simulink model "AOOR"  (R2020a)
settings: Solver=FixedStepAuto  StartTime=0.0  StopTime=60  FixedStep=1e-3  RelTol=1e-3  EnableMultiTasking=on
undefined symbols (not defined in the file): D10, D11, D12, D2, D4, D5, D7, D8, D9, PTA0, PTA2, PTB23, PTB9, PTC3, PTC4, PTD0, PTD2, PTD3
libraries: frdmk64flib x11, dspstat3 x1
settings Model: ExtModeTrigDuration=5  Creator=raymo  LastModifiedBy=raymo
settings OptimizationCC: EnhancedBackFolding=on  PassReuseOutputArgsAs=Individual arguments  ZeroExternalMemoryAtStartup=off  ZeroInternalMemoryAtStartup=off  MaxStackSize=64  OptimizeBlockOrder=speed  DifferentSizesBufferReuse=on  OptimizationCustomize=off  EfficientTunableParamExpr=on
settings DebuggingCC: ParameterTunabilityLossMsg=error
settings HardwareCC: ProdBitPerPointer=32  ProdBitPerSizeT=32  ProdBitPerPtrDiffT=32  ProdLargestAtomicInteger=Long  ProdLargestAtomicFloat=Double  ProdWordSize=32  ProdHWDeviceType=ARM Compatible->ARM Cortex
settings SFSimCC: MATLABDynamicMemAlloc=off
settings RTWCC: SystemTargetFile=ert.tlc  HardwareBoard=NXP FRDM-K64F  TemplateMakefile=ert_default_tmf  Toolchain=GNU Tools for ARM Embedded Processors
settings CodeAppCC: ForceParamTrailComments=on  IgnoreCustomStorageClasses=off  OperatorAnnotations=on  SimulinkDataObjDesc=on  SFDataObjDesc=on  InsertBlockDesc=on

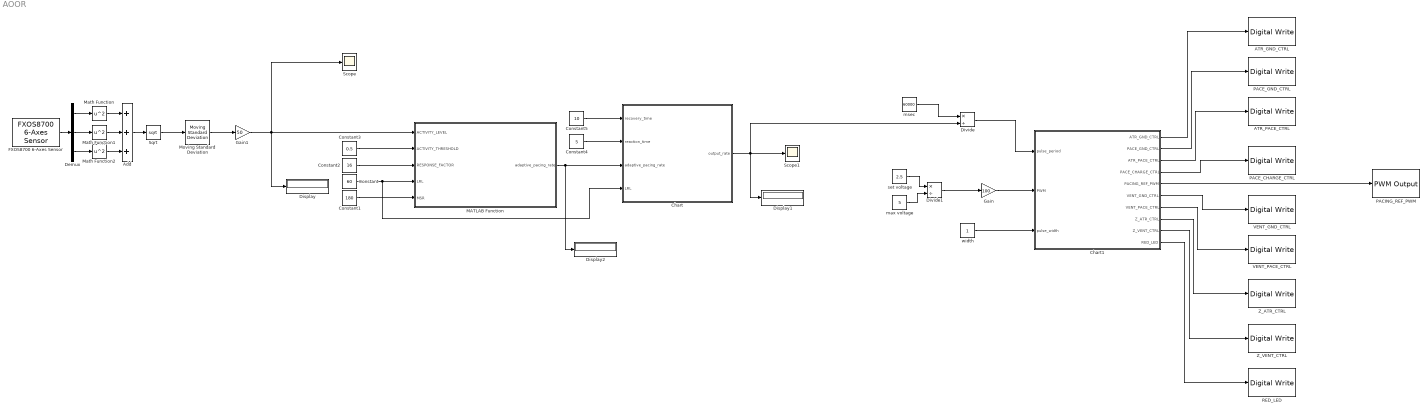
== system AOOR ==
  ATR_GND_CTRL : frdmk64flib/Digital Write  Whichpin=PTD2 (D11)
  ATR_PACE_CTRL : frdmk64flib/Digital Write  Whichpin=PTA0 (D8)
  Add : Sum  Inputs=+++
  Chart : Stateflow chart  TreatAsAtomicUnit=on
  Chart1 : Stateflow chart  TreatAsAtomicUnit=on
  Constant : Constant  Value=60
  Constant1 : Constant  Value=180
  Constant2 : Constant  Value=16
  Constant3 : Constant  Value=0.5
  Constant4 : Constant  Value=5
  Constant5 : Constant  Value=10
  Demux : Demux  Outputs=3
  Display : Display
  Display1 : Display
  Display2 : Display
  Divide : Product  Inputs=*/
  Divide1 : Product  Inputs=*/
  FXOS8700 6-Axes Sensor : frdmk64flib/FXOS8700 6-Axes Sensor  Activesensor=Accelerometer only  ODR=800Hz  HybridODR=400Hz  Accelfullrange=-4g to +4g  SampleTime=-1
  Gain : Gain  Gain=100
  Gain1 : Gain  Gain=50
  MATLAB Function : MATLAB Function  TreatAsAtomicUnit=on
  Math Function : Math  Operator=square  SaturateOnIntegerOverflow=on
  Math Function1 : Math  Operator=square  SaturateOnIntegerOverflow=on
  Math Function2 : Math  Operator=square  SaturateOnIntegerOverflow=on
  Moving Standard Deviation : dspstat3/Moving Standard Deviation  Method=Sliding window  ForgettingFactorPort=off  SpecifyWindowLength=on  WindowLength=4  ForgettingFactor=0.9  SimulateUsing=Code generation
      settings: SourceProductBaseCode=DS
  PACE_CHARGE_CTRL : frdmk64flib/Digital Write  Whichpin=PTB9 (D2)
  PACE_GND_CTRL : frdmk64flib/Digital Write  Whichpin=PTD0 (D10)
  PACING_REF_PWM : frdmk64flib/PWM Output  Whichpin=PTA2 (D5)  InitialFrequency=2000  InitialDutyCycle=50
  RED_LED : frdmk64flib/Digital Write  Whichpin=RED_LED
  Scope : Scope
  Scope1 : Scope
  Sqrt : Sqrt  SaturateOnIntegerOverflow=on
  VENT_GND_CTRL : frdmk64flib/Digital Write  Whichpin=PTD3 (D12)
  VENT_PACE_CTRL : frdmk64flib/Digital Write  Whichpin=PTC4 (D9)
  Z_ATR_CTRL : frdmk64flib/Digital Write  Whichpin=PTB23 (D4)
  Z_VENT_CTRL : frdmk64flib/Digital Write  Whichpin=PTC3 (D7)
  max voltage : Constant  Value=5
  msec : Constant  Value=60000
  set voltage : Constant  Value=2.5
  width : Constant
  wires:
  Math Function1/1 -> Add/2
  Add/1 -> Sqrt/1
  Demux/1 -> Math Function/1
  Demux/3 -> Math Function2/1
  Math Function2/1 -> Add/3
  Sqrt/1 -> Moving Standard Deviation/1
  Math Function/1 -> Add/1
  Demux/2 -> Math Function1/1
  FXOS8700 6-Axes Sensor/1 -> Demux/1
  MATLAB Function/1(adaptive_pacing_rate) -> Chart/3(adaptive_pacing_rate), Display2/1
  Constant/1 -> Chart/4(LRL), MATLAB Function/4(LRL)
  Constant1/1 -> MATLAB Function/5(MSR)
  Constant2/1 -> MATLAB Function/3(RESPONSE_FACTOR)
  Constant3/1 -> MATLAB Function/2(ACTIVITY_THRESHOLD)
  Constant5/1 -> Chart/1(recovery_time)
  Constant4/1 -> Chart/2(reaction_time)
  Chart/1(output_rate) -> Divide/2, Display1/1, Scope1/1
  Divide/1 -> Chart1/1(pulse_period)
  set voltage/1 -> Divide1/1
  Chart1/9(Z_VENT_CTRL) -> Z_VENT_CTRL/1
  Chart1/1(ATR_GND_CTRL) -> ATR_GND_CTRL/1
  Chart1/10(RED_LED) -> RED_LED/1
  width/1 -> Chart1/3(pulse_width)
  Chart1/3(ATR_PACE_CTRL) -> ATR_PACE_CTRL/1
  msec/1 -> Divide/1
  Chart1/4(PACE_CHARGE_CTRL) -> PACE_CHARGE_CTRL/1
  Chart1/6(VENT_GND_CTRL) -> VENT_GND_CTRL/1
  max voltage/1 -> Divide1/2
  Chart1/5(PACING_REF_PWM) -> PACING_REF_PWM/1
  Gain/1 -> Chart1/2(PWM)
  Chart1/7(VENT_PACE_CTRL) -> VENT_PACE_CTRL/1
  Chart1/8(Z_ATR_CTRL) -> Z_ATR_CTRL/1
  Divide1/1 -> Gain/1
  Chart1/2(PACE_GND_CTRL) -> PACE_GND_CTRL/1
  Moving Standard Deviation/1 -> Gain1/1
  Gain1/1 -> Scope/1, Display/1, MATLAB Function/1(ACTIVITY_LEVEL)

== stateflow chart AOOR/Chart1 ==
  state ChargeDishcharge
    entry:
    %C22
    ATR_PACE_CTRL = false;
    VENT_PACE_CTRL = false;
    PACING_REF_PWM = PWM;
    PACE_CHARGE_CTRL = true;
    %C21
    PACE_GND_CTRL = true;
    VENT_PACE_CTRL = false;
    Z_ATR_CTRL = false;
    Z_VENT_CTRL = false;
    ATR_GND_CTRL = true;
    VENT_GND_CTRL = false;
    %RED LED
    RED_LED = false;
  state AVpacing
    entry:
    PACE_CHARGE_CTRL = false;
    PACE_GND_CTRL = true;
    ATR_PACE_CTRL = true;
    ATR_GND_CTRL = false;
    Z_ATR_CTRL = false;
    Z_VENT_CTRL = false;
    VENT_GND_CTRL = false;
    VENT_PACE_CTRL = false;
    PACING_REF_PWM = PWM;
    RED_LED = true;
  (default) -> ChargeDishcharge
  AVpacing -> ChargeDishcharge : [after(pulse_width, msec)]
  ChargeDishcharge -> AVpacing : [after(pulse_period-pulse_width, msec)]
  data: ATR_GND_CTRL output; PACE_GND_CTRL output; ATR_PACE_CTRL output; PACE_CHARGE_CTRL output; PACING_REF_PWM output; VENT_GND_CTRL output; VENT_PACE_CTRL output; Z_ATR_CTRL output; Z_VENT_CTRL output; pulse_period input; PWM input; pulse_width input; RED_LED output

== matlab function AOOR/MATLAB Function ==
  data: ACTIVITY_LEVEL input; adaptive_pacing_rate output; ACTIVITY_THRESHOLD input; RESPONSE_FACTOR input; LRL input; MSR input
function adaptive_pacing_rate = fcn(ACTIVITY_LEVEL, ACTIVITY_THRESHOLD, RESPONSE_FACTOR, LRL , MSR)
    if ACTIVITY_LEVEL <= ACTIVITY_THRESHOLD
        adaptive_pacing_rate = LRL; 
    else
        slope = 2.5*RESPONSE_FACTOR;
        b = LRL - (slope*ACTIVITY_THRESHOLD);
        linear_rate_response = (slope*ACTIVITY_LEVEL) + b;
        if(linear_rate_response >= MSR)
           adaptive_pacing_rate = MSR;
        else
            adaptive_pacing_rate = linear_rate_response;
        end
    end
end

== stateflow chart AOOR/Chart ==
  state IDLE
    entry:
    output_rate = LRL;
  state INIT
    entry:
    %The slope of the time response curves
    step_up = abs((adaptive_pacing_rate - output_rate)/reaction_time);
    step_down = abs((adaptive_pacing_rate - output_rate)/recovery_time);
  state STEP_DOWN
    entry:
    output_rate = output_rate - step_down;
  state STEP_UP
    entry:
    output_rate = output_rate + step_up;
  (default) -> IDLE
  IDLE -> INIT
  INIT -> STEP_UP [order 1] : [output_rate < adaptive_pacing_rate]
  INIT -> STEP_DOWN [order 2] : [output_rate > adaptive_pacing_rate]
  STEP_UP -> INIT : [after(1000,msec)]
  STEP_DOWN -> INIT : [after(1000,msec)]
  data: output_rate output; recovery_time input; reaction_time input; adaptive_pacing_rate input; LRL input; step_up local; step_down local
